simulink model "Alarm_System"  (R2018a)
settings: Solver=FixedStepDiscrete  StartTime=0.0  StopTime=10.0  RelTol=1e-3
settings Model: Creator=Moataz  LastModifiedBy=Moataz
settings OptimizationCC: DefaultParameterBehavior=Inlined  EnhancedBackFolding=on  PassReuseOutputArgsAs=Individual arguments  OptimizeBlockOrder=speed  DifferentSizesBufferReuse=on  OptimizationCustomize=off
settings DebuggingCC: ParameterTunabilityLossMsg=error
settings SFSimCC: MATLABDynamicMemAlloc=off
settings SFSimCC: SimCustomHeaderCode=|
  | #include "LED.h"
  | #include "Switch.h"
  | #include	"Buzzer.h"
  | #include	"STD_TYPES.h"
  | #include	"BIT_MATH.h"
  | #include	"Dio_interface.h"
  | #include	"Dio_private.h"
  | #include	"ADC_interface.h"
  | #include	"ADC_Configuration.h"
settings SFSimCC: SimUserSources=|
  | LED.c
  | Buzzer.c
  | Switch.c
  | Dio_program.c
  | ADC_Program.c
settings RTWCC: SystemTargetFile=ert.tlc  GenCodeOnly=on  TemplateMakefile=ert_default_tmf  GenerateReport=on  RTWUseSimCustomCode=on  IncludeHyperlinkInReport=on  LaunchReport=on  GenerateTraceInfo=on  GenerateTraceReport=on  GenerateTraceReportSl=on  GenerateTraceReportSf=on  GenerateTraceReportEml=on
settings RTWCC: CustomHeaderCode=|
  | #include "LED.h"
  | #include "Switch.h"
  | #include	"Buzzer.h"
  | #include	"STD_TYPES.h"
  | #include	"BIT_MATH.h"
  | #include	"Dio_interface.h"
  | #include	"Dio_private.h"
  | #include	"ADC_interface.h"
  | #include	"ADC_Configuration.h"
settings RTWCC: CustomSource=|
  | LED.c
  | Buzzer.c
  | Switch.c
  | Dio_program.c
  | ADC_Program.c
settings CodeAppCC: ForceParamTrailComments=on  IgnoreCustomStorageClasses=off  OperatorAnnotations=on  SimulinkDataObjDesc=on  SFDataObjDesc=on  InsertBlockDesc=on
settings ERTTargetCC: TargetLangStandard=C99 (ISO)  GenerateSampleERTMain=on  InlinedParameterPlacement=NonHierarchical  ERTCustomFileTemplate=example_file_process.tlc

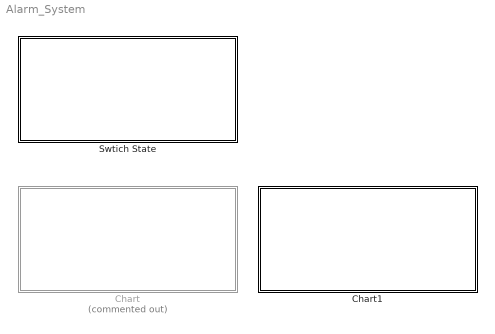
== system Alarm_System ==
  Chart : Stateflow chart  Commented=on  TreatAsAtomicUnit=on
  Chart1 : Stateflow chart  TreatAsAtomicUnit=on
  Swtich State : Stateflow chart  TreatAsAtomicUnit=on

== stateflow chart Alarm_System/Swtich State ==
  (default) -> (junction 178) : {Read_Switch = ReadSwitch(SWITCH_1);}
  (junction 178) -> (junction 179) [order 1] : [Read_Switch==1]
  (junction 179) -> (junction 185) : {Led_TurnOn(LED_GREEN);}
  (junction 178) -> (junction 183) [order 2] : {Led_TurnOff(LED_GREEN);}
  (junction 185) -> (junction 183)
  (junction 183) -> (junction 184)
  data: Read_Switch local boolean

== stateflow chart Alarm_System/Chart ==
  state Read_Temp
    en:
    Analog_Value=ADC_Read(ADC_CHANNEL);
    Digital_Value = Analog_Value * 5000 / 1024;
    Temperature = Digital_Value / 10;
    du:
    ex:
  state Alarm
    (default) -> (junction 97)
    (junction 97) -> (junction 98) [order 1] : [Temperature>=80]
    (junction 97) -> (junction 99) [order 2] : {BuzzerOff();
        | Led_TurnOff(LED_RED);}
    (junction 98) -> (junction 100) : {BuzzerOn();
        | Led_TurnOn(LED_RED);}
    (junction 100) -> (junction 99)
    (junction 99) -> (junction 101)
  (default) -> Read_Temp
  Read_Temp -> Alarm : [Temperature !=0]
  data: Read_Switch local boolean; Switch_Pressed local boolean; Analog_Value local double; Digital_Value local double; Temperature local double

== stateflow chart Alarm_System/Chart1 ==
  state Read_Temp
    en:
    Analog_Value=ADC_Read(ADC_CHANNEL);
    Digital_Value = Analog_Value * 5000 / 1024;
    Temperature = Digital_Value / 10;
    du:
    ex:
  (default) -> Read_Temp
  Read_Temp -> (junction 119)
  (junction 119) -> (junction 120) [order 1] : [Temperature>=80]
  (junction 119) -> (junction 121) [order 2] : {BuzzerOff();
      | Led_TurnOff(LED_RED);}
  (junction 120) -> (junction 127) : {BuzzerOn();
      | Led_TurnOn(LED_RED);}
  (junction 127) -> (junction 121)
  (junction 121) -> (junction 126)
  data: Read_Switch local boolean; Switch_Pressed local boolean; Analog_Value local double; Digital_Value local double; Temperature local double
